simulink model "AutomotiveSystem_ABS"  (R2020b)
settings: Solver=VariableStepAuto  StartTime=0.0  StopTime=25  RelTol=1e-3
PostLoadFcn:
  | I=5;
  | Kf=1;
  | PBmax=1500;
  | Rr=1.25;
  | TB=0.01;
  | ctrl=1;
  | g=32.18;
  | m=50;
  | v0=88;
  | mu=[0 0.4 0.8 0.97 1 0.98 0.96 0.94 0.92 0.9 0.88 0.855 0.83 0.81 0.79 0.77 0.75 0.73 0.72 0.71 0.7]
  | slip=[0 0.05 0.1 0.15000000000000002 0.2 0.25 0.30000000000000004 0.35000000000000003 0.4 0.45 0.5 0.55 0.6 0.64999999999999991 0.7 0.75 0.8 0.85 0.9 0.95 1]
undefined symbols (not defined in the file or in its folder): sigbuilder_block
settings Model: DataDictionary=ABS_dict.sldd  Creator=DELL  LastModifiedBy=DELL

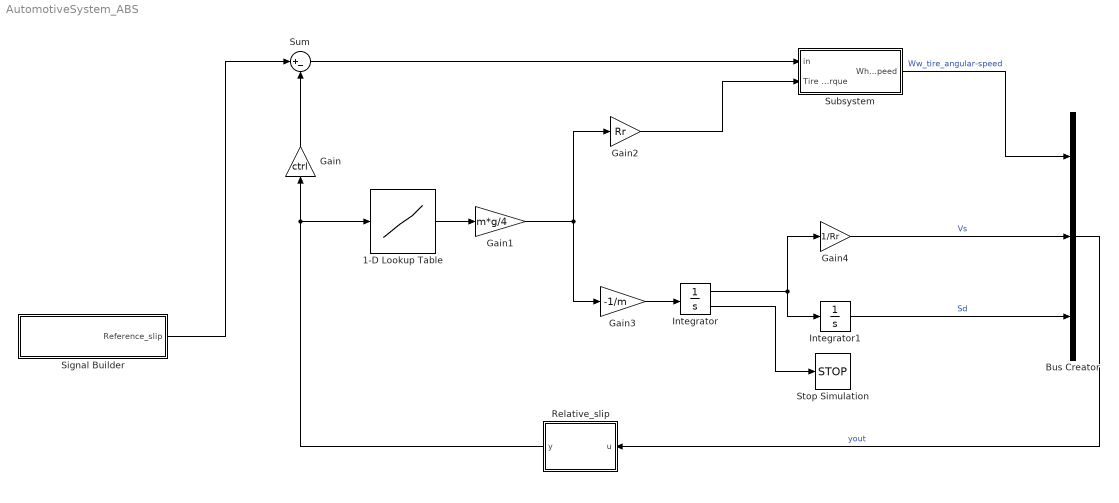
== system AutomotiveSystem_ABS ==
  1-D Lookup Table : Lookup_n-D  NumberOfTableDimensions=1  BreakpointsForDimension1=slip  Table=mu  InternalRulePriority=Speed  RndMeth=Simplest  InputSameDT=on
  Bus Creator : BusCreator  Inputs=3
  Gain : Gain  Gain=ctrl
  Gain1 : Gain  Gain=m*g/4
  Gain2 : Gain  Gain=Rr
  Gain3 : Gain  Gain=-1/m
  Gain4 : Gain  Gain=1/Rr
  Integrator : Integrator  InitialCondition=v0  LimitOutput=on  UpperSaturationLimit=5000  LowerSaturationLimit=0  ShowSaturationPort=on
  Integrator1 : Integrator
  Relative_slip : MATLAB Function  TreatAsAtomicUnit=on
  Signal Builder : Subsystem  Tag=STV Subsys  LoadFcn=sigbuilder_block('load');  StartFcn=sigbuilder_block('start');  StopFcn=sigbuilder_block('stop');  ClipboardFcn=sigbuilder_block('clipboard');  mask(Sigbuilder block){tuvar=[0:10]}
      mask help: Simulink:masks:SigbuilderBlock_MD
      mask init:
      | if ~strcmp(get_param(bdroot(gcbh),'SimulationStatus'),'stopped') tuvar = sigbuilder_block('maskInit'); end
      settings: CopyFcn=sigbuilder_block('copy');  DeleteFcn=sigbuilder_block('delete');  ModelCloseFcn=sigbuilder_block('modelClose');  PreSaveFcn=sigbuilder_block('preSave');  PauseFcn=sigbuilder_block('pause');  ContinueFcn=sigbuilder_block('continue');  NameChangeFcn=sigbuilder_block('namechange');  OpenFcn=sigbuilder_block('open',[437.6 199.2 550.4 400 ]);  CloseFcn=sigbuilder_block('close');
      mask Display: plot(0, 0, 100, 100,[2, 2, 32, 32, 2], [68, 8, 8, 68, 68],[32, 2], [38, 38], [32, 19, 2],[53, 60, 44], [32, 17, 17, 2],[16, 16, 31, 31]);txt = getActiveGroup(gcbh);text(2, 100, txt,'verticalAlignment', 'top');
  Stop Simulation : Stop
  Subsystem : Subsystem
  Sum : Sum  Inputs=|+-
  wires:
  Gain/1 -> Sum/2
  Sum/1 -> Subsystem/1(in)
  1-D Lookup Table/1 -> Gain1/1
  Gain1/1 -> Gain3/1, Gain2/1
  Gain3/1 -> Integrator/1
  Integrator/1 -> Integrator1/1, Gain4/1
  Integrator/2 -> Stop Simulation/1
  Gain2/1 -> Subsystem/2(Tire Torque)
  Integrator1/1 -> Bus Creator/3  "Sd"
  Subsystem/1(Wheel_speed) -> Bus Creator/1  "Ww_tire_angular-speed"
  Gain4/1 -> Bus Creator/2  "Vs"
  Bus Creator/1 -> Relative_slip/1(u)  "yout"
  Relative_slip/1(y) -> 1-D Lookup Table/1, Gain/1
  Signal Builder/1(Reference_slip) -> Sum/1

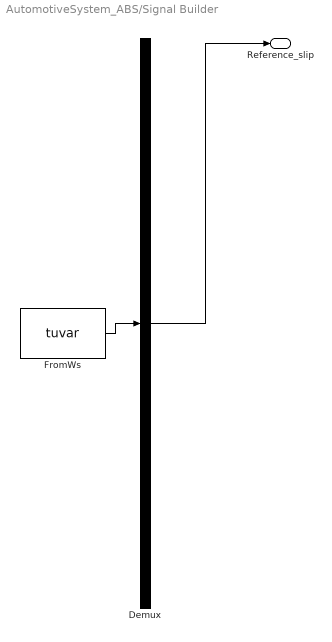
== system AutomotiveSystem_ABS/Signal Builder ==
  Demux : Demux  Tag=STV Demux  Outputs=1
      settings: DisplayOption=none
  FromWs : FromWorkspace  Tag=STV FromWs  VariableName=tuvar
      SigBuilderData=|
      | common.afterFinalStr = 'Extrapolate'
      | common.sampleTime = 0
      | dataSet.timeRange = [0 10]
      | dataSet.name = 'Group 1'
      | sbobj.Groups.Name = 'Group 1'
      | sbobj.Groups.Signals.Name = 'Reference_slip'
      | sbobj.Groups.Signals.XData = [0 4 10]
      | sbobj.Groups.Signals.YData = [0.2 0.2 0.2]
  Reference_slip : Outport  Tag=STV Outport
  wires:
  Demux/1 -> Reference_slip/1
  FromWs/1 -> Demux/1

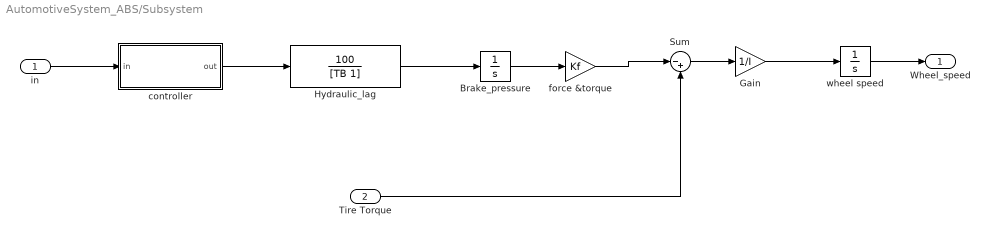
== system AutomotiveSystem_ABS/Subsystem ==
  in : Inport
  Tire Torque : Inport  Port=2
  Brake_pressure : Integrator  LimitOutput=on  UpperSaturationLimit=PBmax  LowerSaturationLimit=0
  Gain : Gain  Gain=1/I
  Hydraulic_lag : TransferFcn  Numerator=100  Denominator=[TB 1]
  Sum : Sum  Inputs=|-+
  controller : Subsystem
  force &torque : Gain  Gain=Kf
  wheel speed : Integrator  InitialCondition=v0/Rr  LimitOutput=on  UpperSaturationLimit=1000  LowerSaturationLimit=0
  Wheel_speed : Outport
  wires:
  in/1 -> controller/1(in)
  controller/1(out) -> Hydraulic_lag/1
  Hydraulic_lag/1 -> Brake_pressure/1
  Brake_pressure/1 -> force &torque/1
  force &torque/1 -> Sum/1
  Tire Torque/1 -> Sum/2
  Sum/1 -> Gain/1
  wheel speed/1 -> Wheel_speed/1
  Gain/1 -> wheel speed/1

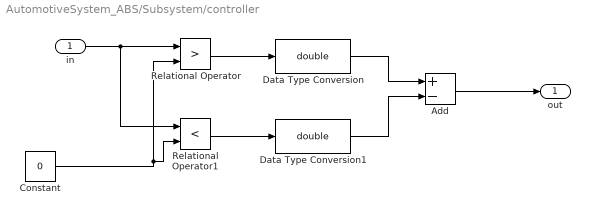
== system AutomotiveSystem_ABS/Subsystem/controller ==
  in : Inport
  Add : Sum  Inputs=+-
  Constant : Constant  Value=0
  Data Type Conversion : DataTypeConversion  OutDataTypeStr=double
  Data Type Conversion1 : DataTypeConversion  OutDataTypeStr=double
  Relational Operator : RelationalOperator  Operator=>  OutDataTypeStr=boolean  RndMeth=Simplest
  Relational Operator1 : RelationalOperator  Operator=<  OutDataTypeStr=boolean  RndMeth=Simplest
  out : Outport
  wires:
  in/1 -> Relational Operator1/1, Relational Operator/1
  Relational Operator/1 -> Data Type Conversion/1
  Relational Operator1/1 -> Data Type Conversion1/1
  Data Type Conversion/1 -> Add/1
  Data Type Conversion1/1 -> Add/2
  Add/1 -> out/1
  Constant/1 -> Relational Operator/2, Relational Operator1/2

== matlab function AutomotiveSystem_ABS/Relative_slip ==
  data: u input; y output
function y = fcn(u)

y = 1.0-u(1)/(u(2)+(u(2)==0)*eps);
